simulink model "TRAS_controller_"  (R2024b)
settings: Solver=FixedStepAuto  StartTime=0.0  StopTime=stop_time  FixedStep=sampling_time  RelTol=1e-3
values from neighbouring files (symbols this model uses):
  A = 0.0552    [momentsOfInertia.m]
  B = 0.0599    [momentsOfInertia.m]
  C = 0.0084    [momentsOfInertia.m]
  D = (mmr + mms + mm / 3) * lm^2 + (mtr + mts + mt / 3) * lt^2    (= 0.0224143186667)    [momentsOfInertia.m]
  derivative_pole_tc = 2 * sampling_time    (= 0.02)    [TRAS_closed_loop.m]
  F = mms * rms^2 + mts * rts^2    (= 0.002355075)    [momentsOfInertia.m]
  g = 9.81    [TRAS_closed_loop.m]    (also in TRAS_controller.m; TRAS_process.m)
  Jv = D + E + F    (= 0.0253918936667)    [momentsOfInertia.m]
  kd = 2 * zeta * wn + pole    (= 8.88888888889)    [TRAS_closed_loop.m]    (also in TRAS_controller.m = 4)
  Kh = [-Kdecline / 4000^2, 0, Kpeak]    [thrustForcesDependencies.m]
  ki = pole * wn^2    (= 7.80368846212)    [TRAS_closed_loop.m]
  ki_inner = wn_inner^2    (= 1849.9248468)    [TRAS_closed_loop.m]
  kp = wn^2 + 2 * zeta * wn * pole    (= 15.890260631)    [TRAS_closed_loop.m]    (also in TRAS_controller.m = 4)
  kp_inner = 2 * zeta_inner * wn_inner    (= 53.3333333333)    [TRAS_closed_loop.m]
  Kv = [-Kdecline / 4000^2, 0, Kpeak]    [thrustForcesDependencies.m]
  L = (mmr + mms + mm / 4) * lm^2 + (mtr + mts + mt / 4) * lt^2 - mcb * lcb^2 - mb / 4 * lb^2    (= 0.021593306)    [momentsOfInertia.m]
  lm = 0.202    [momentsOfInertia.m]
  lt = 0.216    [momentsOfInertia.m]
  Th = [-Tdecline / 4000^2, 0, Tpeak]    [thrustForcesDependencies.m]
  Tv = [-Tdecline / 4000^2, 0, Tpeak]    [thrustForcesDependencies.m]
  x_grid = linspace(-4000, 4000, 1e4)    [TRAS_closed_loop.m]    (also in TRAS_controller.m = linspace(-1, 1, 1e5))
  y_grid_h = polyval(Fh, x_grid)    [TRAS_closed_loop.m]    (also in TRAS_controller.m = polyval(Fh_of_u2, x_grid))
  y_grid_v = polyval(Fv, x_grid)    [TRAS_closed_loop.m]    (also in TRAS_controller.m = polyval(Fv_of_u1, x_grid))
settings Model: Creator=Codrin  LastModifiedBy=Codrin

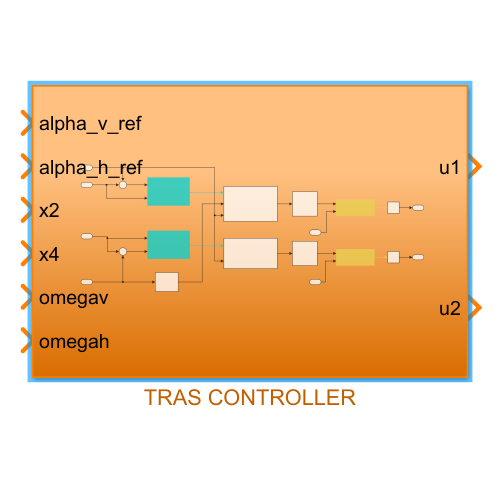
[thumbnail: Simulink's stored preview of the top-level diagram]
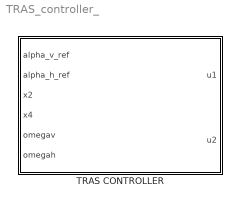
== system TRAS_controller_ ==
  TRAS CONTROLLER : Subsystem

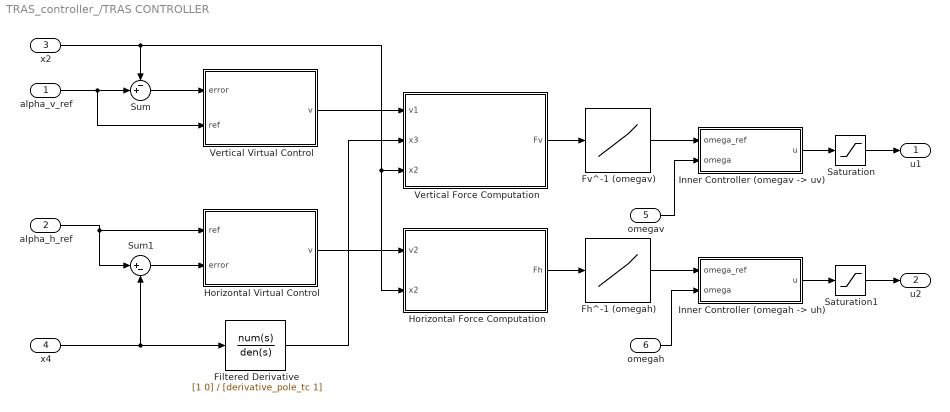
== system TRAS_controller_/TRAS CONTROLLER ==
  alpha_v_ref : Inport
  alpha_h_ref : Inport  Port=2
  x2 : Inport  Port=3
  x4 : Inport  Port=4
  omegav : Inport  Port=5
  omegah : Inport  Port=6
  Fh^-1 (omegah) : Lookup_n-D  NumberOfTableDimensions=1  BreakpointsForDimension1=y_grid_h  Table=x_grid  ExtrapMethod=Clip  InternalRulePriority=Speed  RndMeth=Simplest
  Filtered Derivative : TransferFcn  Numerator=[1 0]  Denominator=[derivative_pole_tc 1]
  Fv^-1 (omegav) : Lookup_n-D  NumberOfTableDimensions=1  BreakpointsForDimension1=y_grid_v  Table=x_grid  InterpMethod=Cubic spline  ExtrapMethod=Clip  InternalRulePriority=Speed  RndMeth=Simplest
  Horizontal Force Computation : MATLAB Function  TreatAsAtomicUnit=on
  Horizontal Virtual Control : Subsystem
  "Inner Controller (omegah -> uh)" : Subsystem
  "Inner Controller (omegav -> uv)" : Subsystem
  Saturation : Saturate  UpperLimit=0.98  LowerLimit=-0.98
  Saturation1 : Saturate  UpperLimit=0.98  LowerLimit=-0.98
  Sum : Sum  Inputs=-+|
  Sum1 : Sum  Inputs=|+-
  Vertical Force Computation : MATLAB Function  TreatAsAtomicUnit=on
  Vertical Virtual Control : Subsystem
  u1 : Outport
  u2 : Outport  Port=2
  wires:
  Filtered Derivative/1 -> Vertical Force Computation/2(x3)
  Vertical Virtual Control/1(v) -> Vertical Force Computation/1(v1)
  x2/1 -> Horizontal Force Computation/2(x2), Vertical Force Computation/3(x2), Sum/1
  Horizontal Virtual Control/1(v) -> Horizontal Force Computation/1(v2)
  Saturation/1 -> u1/1
  x4/1 -> Sum1/2, Filtered Derivative/1
  alpha_v_ref/1 -> Vertical Virtual Control/2(ref), Sum/2
  alpha_h_ref/1 -> Horizontal Virtual Control/1(ref), Sum1/1
  Sum1/1 -> Horizontal Virtual Control/2(error)
  "Inner Controller (omegav -> uv)"/1(u) -> Saturation/1
  omegav/1 -> "Inner Controller (omegav -> uv)"/2(omega)
  "Inner Controller (omegah -> uh)"/1(u) -> Saturation1/1
  omegah/1 -> "Inner Controller (omegah -> uh)"/2(omega)
  Sum/1 -> Vertical Virtual Control/1(error)
  Vertical Force Computation/1(Fv) -> Fv^-1 (omegav)/1
  Horizontal Force Computation/1(Fh) -> Fh^-1 (omegah)/1
  Saturation1/1 -> u2/1
  Fh^-1 (omegah)/1 -> "Inner Controller (omegah -> uh)"/1(omega_ref)
  Fv^-1 (omegav)/1 -> "Inner Controller (omegav -> uv)"/1(omega_ref)

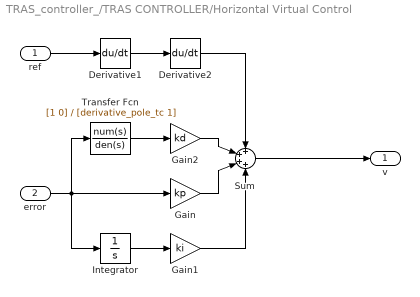
== system TRAS_controller_/TRAS CONTROLLER/Horizontal Virtual Control ==
  ref : Inport
  error : Inport  Port=2
  Derivative1 : Derivative
  Derivative2 : Derivative
  Gain : Gain  Gain=kp
  Gain1 : Gain  Gain=ki
  Gain2 : Gain  Gain=kd
  Integrator : Integrator
  Sum : Sum  Inputs=++++
  Transfer Fcn : TransferFcn  Numerator=[1 0]  Denominator=[derivative_pole_tc 1]
  v : Outport
  wires:
  Sum/1 -> v/1
  Gain1/1 -> Sum/4
  Gain/1 -> Sum/3
  Gain2/1 -> Sum/2
  Derivative2/1 -> Sum/1
  Transfer Fcn/1 -> Gain2/1
  error/1 -> Transfer Fcn/1, Gain/1, Integrator/1
  Derivative1/1 -> Derivative2/1
  ref/1 -> Derivative1/1
  Integrator/1 -> Gain1/1

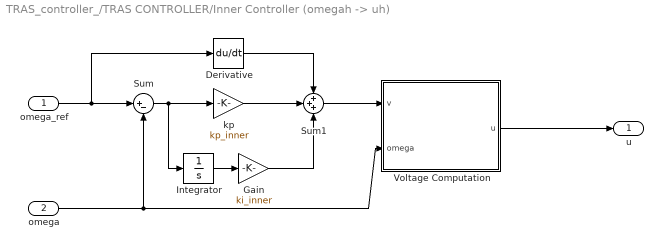
== system TRAS_controller_/TRAS CONTROLLER/Inner Controller (omegah -> uh) ==
  omega_ref : Inport
  omega : Inport  Port=2
  Derivative : Derivative
  Gain : Gain  Gain=ki_inner
  Integrator : Integrator
  Sum : Sum  Inputs=|+-
  Sum1 : Sum  Inputs=+++
  Voltage Computation : MATLAB Function  TreatAsAtomicUnit=on
  kp : Gain  Gain=kp_inner
  u : Outport
  wires:
  Voltage Computation/1(u) -> u/1
  Sum1/1 -> Voltage Computation/1(v)
  Derivative/1 -> Sum1/1
  kp/1 -> Sum1/2
  omega_ref/1 -> Sum/1, Derivative/1
  omega/1 -> Voltage Computation/2(omega), Sum/2
  Gain/1 -> Sum1/3
  Integrator/1 -> Gain/1
  Sum/1 -> Integrator/1, kp/1

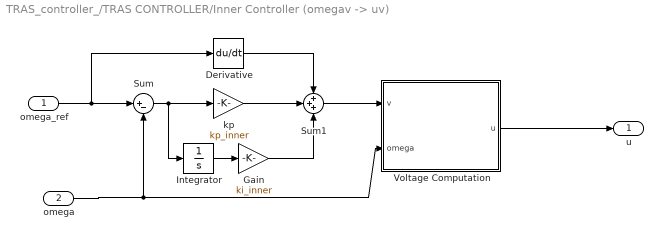
== system TRAS_controller_/TRAS CONTROLLER/Inner Controller (omegav -> uv) ==
  omega_ref : Inport
  omega : Inport  Port=2
  Derivative : Derivative
  Gain : Gain  Gain=ki_inner
  Integrator : Integrator
  Sum : Sum  Inputs=|+-
  Sum1 : Sum  Inputs=+++
  Voltage Computation : MATLAB Function  TreatAsAtomicUnit=on
  kp : Gain  Gain=kp_inner
  u : Outport
  wires:
  omega/1 -> Sum/2, Voltage Computation/2(omega)
  omega_ref/1 -> Derivative/1, Sum/1
  Sum/1 -> Integrator/1, kp/1
  kp/1 -> Sum1/2
  Derivative/1 -> Sum1/1
  Sum1/1 -> Voltage Computation/1(v)
  Voltage Computation/1(u) -> u/1
  Integrator/1 -> Gain/1
  Gain/1 -> Sum1/3

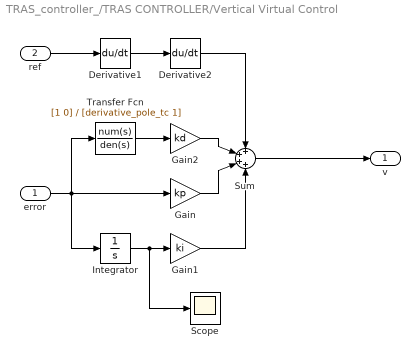
== system TRAS_controller_/TRAS CONTROLLER/Vertical Virtual Control ==
  error : Inport
  ref : Inport  Port=2
  Derivative1 : Derivative
  Derivative2 : Derivative
  Gain : Gain  Gain=kp
  Gain1 : Gain  Gain=ki
  Gain2 : Gain  Gain=kd
  Integrator : Integrator  LimitOutput=on  UpperSaturationLimit=0.2  LowerSaturationLimit=-0.2
  Scope : Scope
  Sum : Sum  Inputs=++++
  Transfer Fcn : TransferFcn  Numerator=[1 0]  Denominator=[derivative_pole_tc 1]
  v : Outport
  wires:
  Integrator/1 -> Scope/1, Gain1/1
  ref/1 -> Derivative1/1
  Derivative1/1 -> Derivative2/1
  error/1 -> Transfer Fcn/1, Integrator/1, Gain/1
  Transfer Fcn/1 -> Gain2/1
  Derivative2/1 -> Sum/1
  Gain2/1 -> Sum/2
  Gain/1 -> Sum/3
  Gain1/1 -> Sum/4
  Sum/1 -> v/1

== matlab function TRAS_controller_/TRAS CONTROLLER/Vertical Force Computation ==
  data: Fv output; v1 input; x3 input; x2 input; Jv parameter; L parameter; g parameter; A parameter; B parameter; C parameter; lm parameter
function Fv = verticalForceComputation(v1, x3, x2, Jv, L, g, A, B, C, lm)

Fv = 1 / lm * (v1 * Jv + x3^2 / 2 * L * sin(2 * x2) - g * ((A-B)*cos(x2) - C*sin(x2)));

== matlab function TRAS_controller_/TRAS CONTROLLER/Horizontal Force Computation ==
  data: v2 input; Fh output; x2 input; lt parameter; D parameter; E parameter; F parameter
function Fh = horizontalForceComputation(v2, x2, lt, D, E, F)

Fh = v2 / (lt * cos(x2)) * (D * cos(x2)^2 + E * sin(x2)^2 + F);

== matlab function TRAS_controller_/TRAS CONTROLLER/Inner Controller (omegav -> uv)/Voltage Computation ==
  data: v input; u output; omega input; Tv parameter; Kv parameter
function u = voltageComputation(v, omega, Tv, Kv)

u = polyval(Tv, omega) / polyval(Kv, omega) * (v + polyval(Tv, omega) * omega);

== matlab function TRAS_controller_/TRAS CONTROLLER/Inner Controller (omegah -> uh)/Voltage Computation ==
  data: v input; u output; omega input; Th parameter; Kh parameter
function u = voltageComputation(v, omega, Th, Kh)

u = polyval(Th, omega) / polyval(Kh, omega) * (v + polyval(Th, omega) * omega);
